simulink model "miniprojectjaaa"  (R2021a)
settings: Solver=VariableStepAuto  StartTime=0.0  StopTime=10  RelTol=1e-3
undefined symbols (not defined in the file or in its folder): Discrete, magnitude, Time
libraries: ctrlSharedLib x3
settings Model: Creator=user  LastModifiedBy=thana

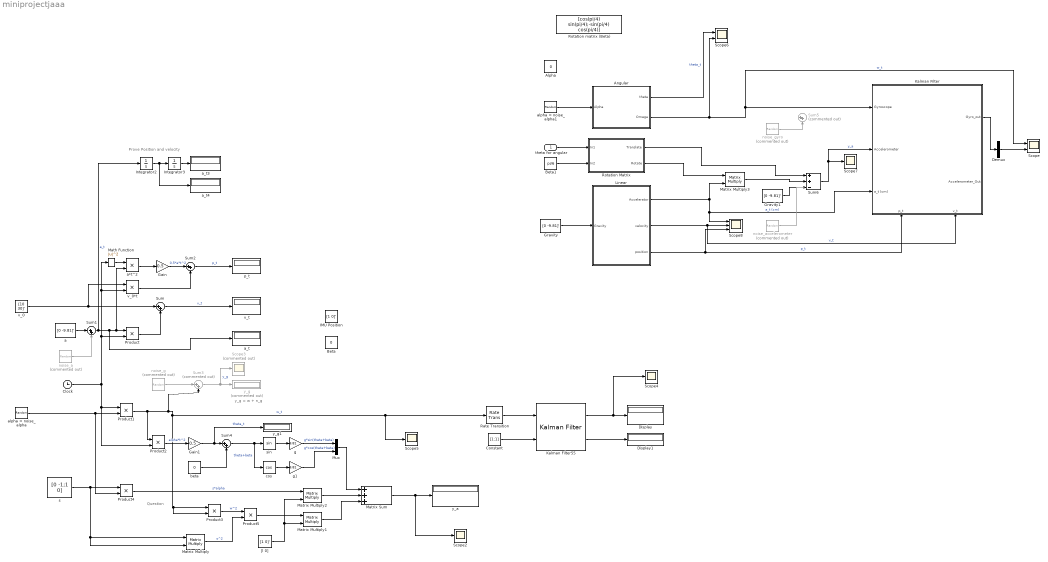
== system miniprojectjaaa ==
  note: Question
  note: Prove Position and velocity
  note: y_g = w + n_g
  theta for angular : Inport
  Alpha : Constant  Value=0
  Angular : Subsystem
  Beta : Constant  Value=0  VectorParams1D=off
  Beta1 : Constant  Value=pi/6
  Clock : Clock
  Constant : Constant  Value=[1;1]  VectorParams1D=off
  Demux : Demux  Outputs=3
  Display : Display
  Display1 : Display
  Gain : Gain  Gain=0.5
  Gain1 : Gain  Gain=0.5
  Gravity : Constant  Value=[0 -9.81]'  VectorParams1D=off
  Gravity1 : Constant  Value=[0 -9.81]'  VectorParams1D=off  SampleTime=0.1
  IMU Position : Constant  Value=[1 0]'  VectorParams1D=off
  Integrator2 : Integrator  InitialCondition=[10;30]
  Integrator3 : Integrator
  Kalman Filter : Subsystem
      settings: PortSchema="{\"entries\":[{\"content\":{\"sides\":[{\"content\":{\"connectorIds\":[\"In1\",\"In2\",\"In3\"]},\"type\":\"ConnectorPlacement.EquallySpacedRectSide\",\"uuid\":\"b91da42b-9c61-4823-9da5-de67facf4bc9\"},{\"content\":{\"connectorIds\":[\"Out1\",\"Out2\"],\"side\":\"RIGHT\"},\"type\":\"ConnectorPlacement.EquallySpacedRectSide\",\"uuid\":\"2be3e4bd-003a-4305-9356-0140a49c88fd\"},{\"content\":{\"connectorIds\":[],\"side\":\"TOP\"},\"type\":\"ConnectorPlacement.EquallySpacedRectSide\",\"uuid\":\"082c92ba-2267-4dcd-8603-51b46770a288\"},{\"content\":{\"connectorIds\":[\"In4\",\"In5\"],\"side\":\"BOTTOM\"},\"type\":\"ConnectorPlacement.EquallySpacedRectSide\",\"uuid\":\"6ce4a481-da86-4ab0-8532-700fe3275410\"}]},\"type\":\"ConnectorPlacement.EquallySpacedConnector\",\"uuid\":\"cf631ac5-4969-4497-82c5-cfc4b2b0c485\"}],\"packageUris\":[\"http://schema.mathworks.com/mf0/Connector/R2020b\"],\"version\":\"1.0\"}"
  Kalman Filter55 : ctrlSharedLib/Kalman Filter  TimeDomain=Discrete-Time  UseCurrentEstimator=on  ModelSource=Individual A, B, C, D matrices  ModelSourceVariable=ss(0.95,1,1,0,1)  A=[1 0.01 ;0 1]  B=[0 0;0 0]  C=[0 1]  D=[0]  NumberOfStates=6  NumberOfInputs=1  NumberOfOutputs=1  InitialEstimateSource=Dialog  X0=0  P0=0.1  UseK=off  UseGH=off  NumberOfProcessNoiseInputs=1  G=[(0.01^2)/2;0.01]  TimeInvariantG=on  H=0  TimeInvariantH=on  Q=[1 0;0 1]  TimeInvariantQ=on  R=[1]  TimeInvariantR=on  N=[1;1]  TimeInvariantN=off  AddInputPort=off  AddEnablePort=off  OutputEstimatedY=on  OutputP=off  Ts=-1
  Linear : Subsystem
  Math Function : Math  Operator=magnitude^2  SaturateOnIntegerOverflow=on
  Matrix Sum : Sum  Inputs=+++
  Matrix Multiply{,1..3} (4 alike) : Product  Multiplication=Matrix(*)
  Mux : Mux  Inputs=2
  Product{,1..5} (6 alike) : Product
  Rate Transition : RateTransition
  Rotation Matrix : Subsystem
  Rotation matrix (Beta) : Constant  Value=[cos(pi/4) sin(pi/4);-sin(pi/4) cos(pi/4)]  VectorParams1D=off
  Scope : Scope  NumInputPorts=2
  Scope{2,4..5,7} (4 alike) : Scope
  Scope3 : Scope  Commented=on
  Scope6 : Scope  NumInputPorts=2
  Scope8 : Scope  NumInputPorts=3
  Sum{,1..2,4} (4 alike) : Sum  Inputs=|++
  Sum3 : Sum  Commented=on  Inputs=|++
  Sum5 : Sum  Commented=on  Inputs=|++
  Sum6 : Sum  Inputs=++-
  "[l 0]" : Constant  Value=[1 0]'  VectorParams1D=off
  a : Constant  Value=[0 -9.81]'  VectorParams1D=off
  a*t^2 : Product
  a_t : Display
  a_t3 : Display
  a_t4 : Display
  alpha = noise_alpha : RandomNumber  Variance=0.01  SampleTime=0.1  VectorParams1D=off
  alpha = noise_alpha1 : RandomNumber  Variance=0.01  SampleTime=0.1
  beta : Constant  Value=0
  cos : Trigonometry  Operator=cos
  g : Gain  Gain=9.81
  g1 : Gain  Gain=9.81
  noise_a : RandomNumber  Commented=on  Mean=[0 0]'  Variance=[0.01 0.01]'  Seed=[0 0]'  SampleTime=0.1
  noise_accelerometer : RandomNumber  Commented=on  Variance=[0.01 0.01]  SampleTime=0.1
  noise_g : RandomNumber  Commented=on  Variance=0.01  SampleTime=0.1
  noise_gyro : RandomNumber  Commented=on  Variance=[0.01]  SampleTime=0.1
  p_t : Display
  s : Constant  Value=[0 -1;1 0]  VectorParams1D=off
  sin : Trigonometry
  v_0 : Constant  Value=[10 30]'  VectorParams1D=off
  v_0*t : Product
  v_t : Display
  y_a : Display
  y_g : Display  Commented=on
  y_g1 : Display
  wires:
  a/1 -> Sum1/1
  noise_a/1 -> Sum1/2
  Sum1/1 -> Integrator2/1, a_t/1, a*t^2/2, Product/1  "a_t"
  Clock/1 -> Product/2, Math Function/1, v_0*t/2, Product2/2, Product1/1
  v_0/1 -> v_0*t/1, Sum/1
  Product/1 -> Sum/2
  Sum/1 -> v_t/1  "v_t"
  v_0*t/1 -> Sum2/2
  Sum2/1 -> p_t/1  "p_t"
  Gain/1 -> Sum2/1  "0.5*a*t^2"
  a*t^2/1 -> Gain/1
  alpha = noise_alpha/1 -> Product4/2, Product1/2
  Product1/1 -> Sum3/2, Scope5/1, Rate Transition/1, Product3/2, Product3/1, Product2/1  "w_t"
  Product2/1 -> Gain1/1  "alpha*t^2"
  Gain1/1 -> y_g1/1, Sum4/1  "theta_t"
  noise_g/1 -> Sum3/1
  Sum3/1 -> Scope3/1, y_g/1  "y_g"
  s/1 -> Product4/1, Matrix Multiply/2, Matrix Multiply/1
  Matrix Multiply1/1 -> Matrix Sum/3
  beta/1 -> Sum4/2
  Sum4/1 -> cos/1, sin/1  "theta+beta"
  sin/1 -> g/1
  cos/1 -> g1/1
  g/1 -> Mux/1  "g*sin(theta+beta)"
  g1/1 -> Mux/2  "g*cos(theta+beta)"
  Mux/1 -> Matrix Sum/1
  Matrix Sum/1 -> Scope2/1, y_a/1
  Matrix Multiply/1 -> Product5/2  "s^2"
  Product5/1 -> Matrix Multiply1/1
  "[l 0]"/1 -> Matrix Multiply2/2, Matrix Multiply1/2
  Product3/1 -> Product5/1  "w^2"
  Product4/1 -> Matrix Multiply2/1  "s*alpha"
  Matrix Multiply2/1 -> Matrix Sum/2
  Kalman Filter55/1 -> Scope4/1, Display/1
  Kalman Filter55/2 -> Display1/1
  Constant/1 -> Kalman Filter55/2
  Rate Transition/1 -> Kalman Filter55/1
  Math Function/1 -> a*t^2/1
  Integrator2/1 -> a_t4/1, Integrator3/1
  Integrator3/1 -> a_t3/1
  Gravity/1 -> Linear/1(Gravity)
  Angular/2(Omega) -> Scope/1, Kalman Filter/1(Gyroscope), Scope6/2  "w_t"
  noise_gyro/1 -> Sum5/2
  Angular/1(theta) -> Scope6/1  "theta_t"
  Linear/1(Accelerator) -> Kalman Filter/3(a_t (cm)), Scope8/1, Matrix Multiply3/2  "a_t (cm)"
  Rotation Matrix/1(Translate) -> Sum6/1
  Matrix Multiply3/1 -> Sum6/2
  Linear/2(velocity) -> Kalman Filter/5(v_t), Scope8/2  "v_t"
  Linear/3(position) -> Kalman Filter/4(p_t), Scope8/3  "p_t"
  Gravity1/1 -> Sum6/3
  Sum6/1 -> Scope7/1, Kalman Filter/2(Accelerometer)  "y_a"
  noise_accelerometer/1 -> ?
  Kalman Filter/1(Gyro_out) -> Demux/1
  alpha = noise_alpha1/1 -> Angular/1(Alpha)
  Demux/2 -> Scope/2
  Rotation Matrix/2(Rotate) -> Matrix Multiply3/1
  Beta1/1 -> Rotation Matrix/2(In2)
  theta for angular/1 -> Rotation Matrix/1(In1)

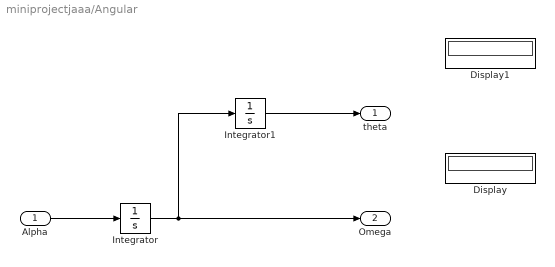
== system miniprojectjaaa/Angular ==
  Alpha : Inport
  Display : Display
  Display1 : Display
  Integrator : Integrator
  Integrator1 : Integrator  InitialCondition=pi/6
  theta : Outport
  Omega : Outport  Port=2
  wires:
  Alpha/1 -> Integrator/1
  Integrator/1 -> Integrator1/1, Omega/1
  Integrator1/1 -> theta/1

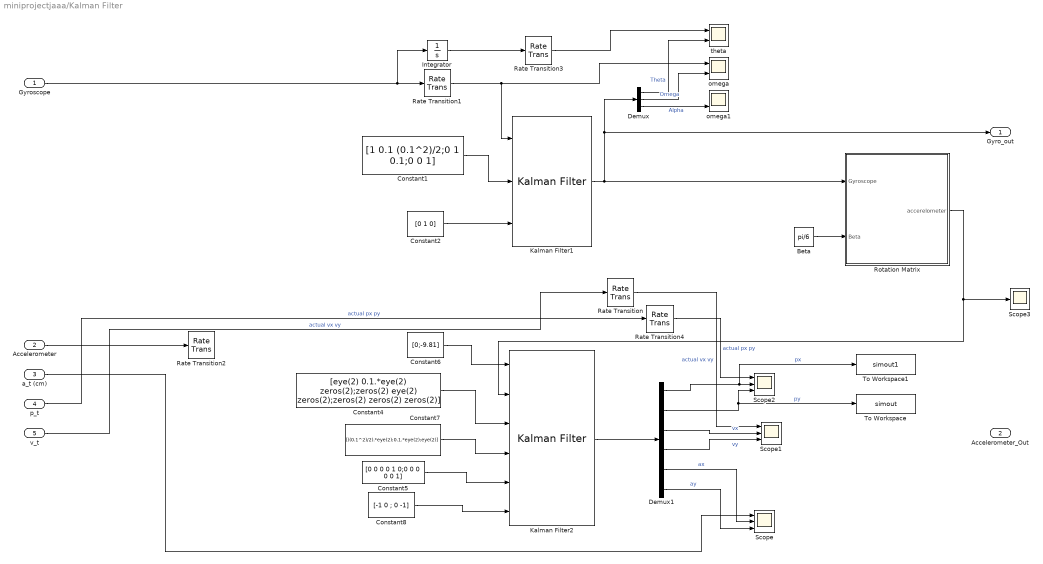
== system miniprojectjaaa/Kalman Filter ==
  Gyroscope : Inport
  Accelerometer : Inport  Port=2
  a_t (cm) : Inport  Port=3
  p_t : Inport  Port=4
  v_t : Inport  Port=5
  Beta : Constant  Value=pi/6
  Constant1 : Constant  Value=[1 0.1 (0.1^2)/2;0 1 0.1;0 0 1]  VectorParams1D=off  SampleTime=0.1
  Constant2 : Constant  Value=[0 1 0]  VectorParams1D=off  SampleTime=0.1
  Constant4 : Constant  Value=[eye(2) 0.1.*eye(2) zeros(2);zeros(2) eye(2) zeros(2);zeros(2) zeros(2) zeros(2)]  VectorParams1D=off  SampleTime=0.1
  Constant5 : Constant  Value=[0 0 0 0 1 0;0 0 0 0 0 1]  VectorParams1D=off  SampleTime=0.1
  Constant6 : Constant  Value=[0;-9.81]  VectorParams1D=off  SampleTime=0.1
  Constant7 : Constant  Value=[((0.1^2)/2).*eye(2);0.1.*eye(2);eye(2)]  VectorParams1D=off  SampleTime=0.1
  Constant8 : Constant  Value=[-1 0 ; 0 -1]  VectorParams1D=off  SampleTime=0.1
  Demux : Demux  Outputs=3
  Demux1 : Demux  Outputs=6
  Integrator : Integrator  InitialCondition=pi/6
  Kalman Filter1 : ctrlSharedLib/Kalman Filter  TimeDomain=Discrete-Time  UseCurrentEstimator=on  ModelSource=Input port  ModelSourceVariable=ss(0.95,1,1,0,1)  A=[1 0.1 0;0 1 0;0 0 1]  B=[0 0;0 0]  C=[0 1 0]  D=[0]  NumberOfStates=3  NumberOfInputs=1  NumberOfOutputs=1  InitialEstimateSource=Dialog  X0=[pi/6 0 0]  P0=0.01  UseK=off  UseGH=on  NumberOfProcessNoiseInputs=1  G=[(0.1^3)/6;(0.1^2)/2;0.1]  TimeInvariantG=on  H=1  TimeInvariantH=on  Q=0.01  TimeInvariantQ=on  R=0.01  TimeInvariantR=on  N=0  TimeInvariantN=on  AddInputPort=off  AddEnablePort=off  OutputEstimatedY=off  OutputP=off  Ts=0.1
  Kalman Filter2 : ctrlSharedLib/Kalman Filter  TimeDomain=Discrete-Time  UseCurrentEstimator=on  ModelSource=Input port  ModelSourceVariable=ss(0.95,1,1,0,1)  A=[1 0.1 0;0 1 0;0 0 1]  B=[0 0;0 0]  C=[0 1 0]  D=[0]  NumberOfStates=6  NumberOfInputs=2  NumberOfOutputs=2  InitialEstimateSource=Dialog  X0=[0 0 5 5 0 0]  P0=0.01  UseK=off  UseGH=on  NumberOfProcessNoiseInputs=1  G=[((0.1^2)/2)*eye(2);0.1*eye(2);eye(2)]  TimeInvariantG=on  H=0  TimeInvariantH=on  Q=0.01  TimeInvariantQ=on  R=0.01  TimeInvariantR=on  N=0  TimeInvariantN=on  AddInputPort=on  AddEnablePort=off  OutputEstimatedY=off  OutputP=off  Ts=0.1
  Rate Transition{,1..4} (5 alike) : RateTransition  OutPortSampleTime=0.1
  Rotation Matrix : Subsystem
  Scope : Scope  NumInputPorts=3
  Scope1 : Scope  NumInputPorts=3
  Scope2 : Scope  NumInputPorts=3
  Scope3 : Scope
  To Workspace : ToWorkspace  VariableName=simout  SaveFormat=Timeseries  SampleTime=-1
  To Workspace1 : ToWorkspace  VariableName=simout1  SaveFormat=Timeseries  SampleTime=-1
  omega : Scope  NumInputPorts=2
  omega1 : Scope  NumInputPorts=2
  theta : Scope  NumInputPorts=2
  Gyro_out : Outport
  Accelerometer_Out : Outport  Port=2
  wires:
  Rate Transition1/1 -> omega/1, Kalman Filter1/1
  Gyroscope/1 -> Integrator/1, Rate Transition1/1
  Constant1/1 -> Kalman Filter1/2
  Constant2/1 -> Kalman Filter1/3
  Accelerometer/1 -> Rate Transition2/1
  Kalman Filter2/1 -> Demux1/1
  Constant4/1 -> Kalman Filter2/3
  Constant6/1 -> Kalman Filter2/1
  Constant7/1 -> Kalman Filter2/4
  Integrator/1 -> Rate Transition3/1
  Rate Transition3/1 -> theta/1
  Kalman Filter1/1 -> Rotation Matrix/1(Gyroscope), Gyro_out/1, Demux/1
  Demux/1 -> theta/2  "Theta"
  Demux/2 -> omega/2  "Omega"
  Rotation Matrix/1(accerelometer) -> Scope3/1, Kalman Filter2/2
  Beta/1 -> Rotation Matrix/2(Beta)
  Constant5/1 -> Kalman Filter2/5
  Constant8/1 -> Kalman Filter2/6
  Demux/3 -> omega1/2  "Alpha"
  Demux1/1 -> To Workspace1/1, Scope2/2  "px"
  Demux1/2 -> Scope2/3, To Workspace/1  "py"
  Demux1/3 -> Scope1/2  "vx"
  Demux1/4 -> Scope1/3  "vy"
  Demux1/5 -> Scope/2  "ax"
  Demux1/6 -> Scope/3  "ay"
  a_t (cm)/1 -> Scope/1
  p_t/1 -> Rate Transition4/1  "actual px py"
  v_t/1 -> Rate Transition/1  "actual vx vy"
  Rate Transition/1 -> Scope1/1  "actual vx vy"
  Rate Transition4/1 -> Scope2/1  "actual px py"

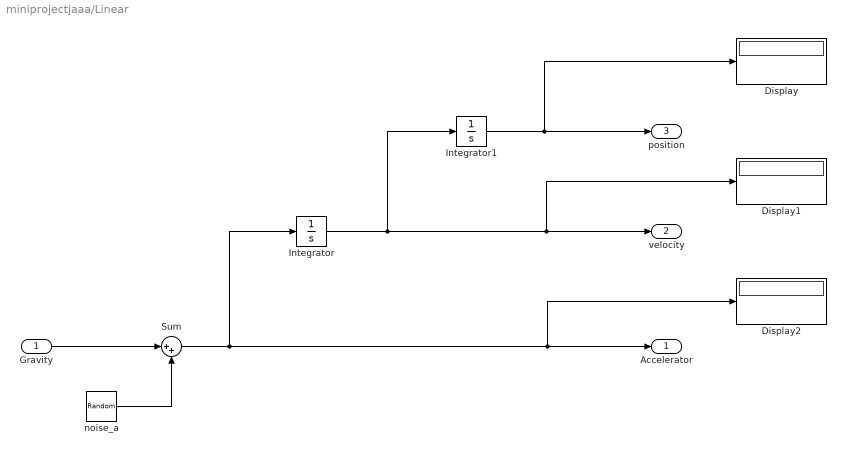
== system miniprojectjaaa/Linear ==
  Gravity : Inport
  Display : Display
  Display1 : Display
  Display2 : Display
  Integrator : Integrator  InitialCondition=[5 5]'
  Integrator1 : Integrator  InitialCondition=[0 0]'
  Sum : Sum  Inputs=|++
  noise_a : RandomNumber  SampleTime=0.1
  Accelerator : Outport
  velocity : Outport  Port=2
  position : Outport  Port=3
  wires:
  Gravity/1 -> Sum/1
  noise_a/1 -> Sum/2
  Sum/1 -> Display2/1, Accelerator/1, Integrator/1
  Integrator/1 -> Integrator1/1, Display1/1, velocity/1
  Integrator1/1 -> Display/1, position/1

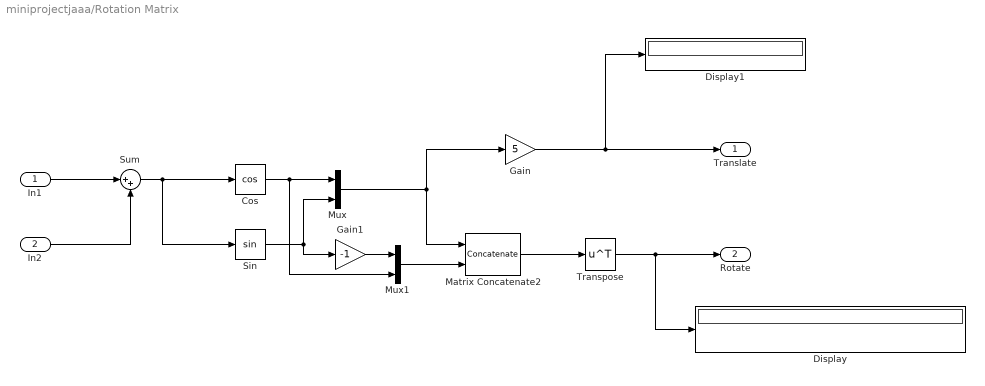
== system miniprojectjaaa/Rotation Matrix ==
  In1 : Inport
  In2 : Inport  Port=2
  Cos : Trigonometry  Operator=cos
  Display : Display
  Display1 : Display
  Gain : Gain  Gain=5
  Gain1 : Gain  Gain=-1
  Matrix Concatenate2 : Concatenate  Mode=Multidimensional array  ConcatenateDimension=2
  Mux : Mux  Inputs=2
  Mux1 : Mux  Inputs=2
  Sin : Trigonometry
  Sum : Sum  Inputs=|++
  Transpose : Math  Operator=transpose  SaturateOnIntegerOverflow=on
  Translate : Outport
  Rotate : Outport  Port=2
  wires:
  Mux/1 -> Gain/1, Matrix Concatenate2/1
  In1/1 -> Sum/1
  Sum/1 -> Sin/1, Cos/1
  Sin/1 -> Gain1/1, Mux/2
  Matrix Concatenate2/1 -> Transpose/1
  Cos/1 -> Mux1/2, Mux/1
  Gain1/1 -> Mux1/1
  Mux1/1 -> Matrix Concatenate2/2
  In2/1 -> Sum/2
  Transpose/1 -> Display/1, Rotate/1
  Gain/1 -> Display1/1, Translate/1

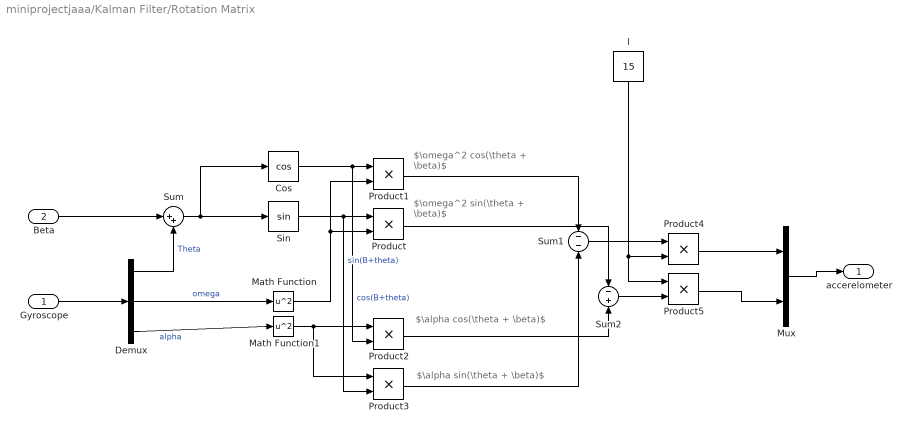
== system miniprojectjaaa/Kalman Filter/Rotation Matrix ==
  note: $\omega^2 sin(\theta + \beta)$
  note: $\omega^2 cos(\theta + \beta)$
  note: $\alpha sin(\theta + \beta)$
  note: $\alpha cos(\theta + \beta)$
  Gyroscope : Inport
  Beta : Inport  Port=2
  Cos : Trigonometry  Operator=cos
  Demux : Demux  Outputs=3
  Math Function : Math  Operator=square  SaturateOnIntegerOverflow=on
  Math Function1 : Math  Operator=square  SaturateOnIntegerOverflow=on
  Mux : Mux  Inputs=2
  Product{,1..5} (6 alike) : Product
  Sin : Trigonometry
  Sum : Sum  Inputs=|++
  Sum1 : Sum  Inputs=--
  Sum2 : Sum  Inputs=-+
  l : Constant  Value=15  VectorParams1D=off  SampleTime=0.1
  accerelometer : Outport
  wires:
  Sum/1 -> Cos/1, Sin/1
  Gyroscope/1 -> Demux/1
  Demux/1 -> Sum/2  "Theta"
  Beta/1 -> Sum/1
  Cos/1 -> Product2/2, Product1/1  "cos(B+theta)"
  Sin/1 -> Product3/2, Product/1  "sin(B+theta)"
  Mux/1 -> accerelometer/1
  Demux/2 -> Math Function/1  "omega"
  Demux/3 -> Math Function1/1  "alpha"
  Math Function/1 -> Product1/2, Product/2
  Product/1 -> Sum2/1
  Product1/1 -> Sum1/1
  Math Function1/1 -> Product3/1, Product2/1
  Product2/1 -> Sum2/2
  Product3/1 -> Sum1/2
  Product4/1 -> Mux/1
  Sum2/1 -> Product5/2
  Sum1/1 -> Product4/1
  l/1 -> Product5/1, Product4/2
  Product5/1 -> Mux/2
